simulink model "deser_simu"  (R2019b)
settings: Solver=VariableStepAuto  StartTime=0.0  StopTime=5000  RelTol=1e-3
InitFcn:
  | %% DSPBuilder Start
  | alt_dspbuilder_update_model(bdroot)
  | %% DSPBuilder End
  | 
  | serializer_init
StartFcn:
  | %% DSPBuilder Start
  | alt_dspbuilder_hdlimport_prepare_for_simulation(bdroot)
  | %% DSPBuilder End
StopFcn:
  | serializer_analysis
libraries: dspsrcs4 x2
settings Model: Creator=vboxuser  LastModifiedBy=vboxuser

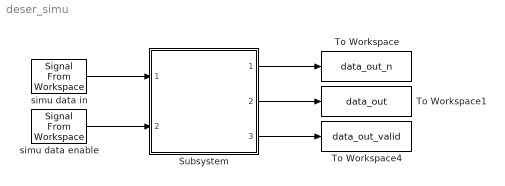
== system deser_simu ==
  Subsystem : Subsystem  ReferencedSubsystem=deser  edge_triggered=off
  To Workspace : ToWorkspace  VariableName=data_out_n  SampleTime=-1
      settings: Save2DSignal=2-D array (concatenate along first dimension)
  To Workspace1 : ToWorkspace  VariableName=data_out  SampleTime=-1
      settings: Save2DSignal=2-D array (concatenate along first dimension)
  To Workspace4 : ToWorkspace  VariableName=data_out_valid  SampleTime=-1
      settings: Save2DSignal=2-D array (concatenate along first dimension)
  simu data enable : dspsrcs4/Signal From Workspace  X=data_en  Ts=1  nsamps=1  OutputAfterFinalValue=Setting to zero  ignoreOrWarnInputAndFrameLengths=off  OutputFrames=off
  simu data in : dspsrcs4/Signal From Workspace  X=data_in  Ts=1  nsamps=1  OutputAfterFinalValue=Setting to zero  ignoreOrWarnInputAndFrameLengths=off  OutputFrames=off
  wires:
  simu data in/1 -> Subsystem/1
  simu data enable/1 -> Subsystem/2
  Subsystem/1 -> To Workspace/1
  Subsystem/2 -> To Workspace1/1
  Subsystem/3 -> To Workspace4/1
